simulink model "Openloop_gendata_2015a"  (Simulink 8.5)
settings: Solver=ode45  SolverMode=SingleTasking  StartTime=0.0  StopTime=10  MaxStep=0.001  RelTol=1e-3
settings Model: Creator=manzand  LastModifiedBy=dieman95  CovMetricSettings=dwe  CovHtmlReporting=off  covSaveCumulativeToWorkspaceVar=off  CovSaveSingleToWorkspaceVar=off  CovExternalEMLEnable=on
settings DataIOCC: LimitDataPoints=off  SaveFormat=Dataset  SignalLoggingSaveFormat=Dataset
settings OptimizationCC: ExpressionDepthLimit=128
settings DebuggingCC: UnderspecifiedInitializationDetection=Simplified  MergeDetectMultiDrivingBlocksExec=error  FcnCallInpInsideContextMsg=EnableAllAsError  StateNameClashWarn=none  SFUnexpectedBacktrackingDiag=error  SFNoUnconditionalDefaultTransitionDiag=error
settings HardwareCC: ProdBitPerPointer=64  ProdLargestAtomicFloat=Float  ProdIntDivRoundTo=Zero  ProdEndianess=LittleEndian  ProdHWDeviceType=Specified
settings ModelReferenceCC: PropagateSignalLabelsOutOfModel=on
settings GRTTargetCC: TargetLangStandard=C99 (ISO)  GeneratePreprocessorConditionals=Use local settings  CombineOutputUpdateFcns=on  GRTInterface=off

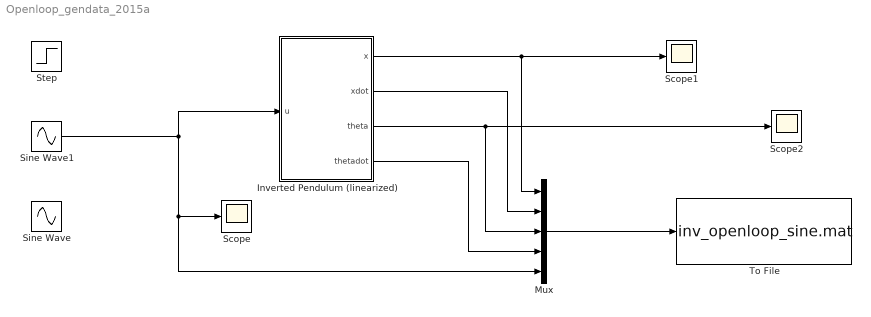
== system Openloop_gendata_2015a ==
  Inverted Pendulum (linearized) : Subsystem
  Mux : Mux  Inputs=5
  Scope : Scope
      settings: TimeRange=auto  MaxDataPoints=5000  SaveToWorkspace=off  SaveName=ScopeData  YMin=-1.25  YMax=1.25  SampleTime=-1
  Scope1 : Scope
      settings: TimeRange=auto  MaxDataPoints=5000  SaveToWorkspace=off  YMin=-49076167611524168.00000  YMax=5452907512391574.00000  SampleTime=-1
  Scope2 : Scope
      settings: TimeRange=auto  MaxDataPoints=5000  SaveToWorkspace=off  SaveName=ScopeData2  YMin=-31802048934758674000.00000  YMax=3533560992750962700.00000  SampleTime=-1
  Sine Wave : Sin  Amplitude=1.4370  Bias=-1.0524  SampleTime=0
  Sine Wave1 : Sin  Amplitude=0.01
  Step : Step  Time=3  SampleTime=0
  To File : ToFile  Filename=inv_openloop_sine.mat  MatrixName=openloop  SampleTime=0.001
      settings: Decimation=2
  wires:
  Sine Wave1/1 -> Inverted Pendulum (linearized)/1(u), Mux/5, Scope/1
  Inverted Pendulum (linearized)/1(x) -> Mux/1, Scope1/1
  Inverted Pendulum (linearized)/3(theta) -> Mux/3, Scope2/1
  Inverted Pendulum (linearized)/2(xdot) -> Mux/2
  Inverted Pendulum (linearized)/4(thetadot) -> Mux/4
  Mux/1 -> To File/1

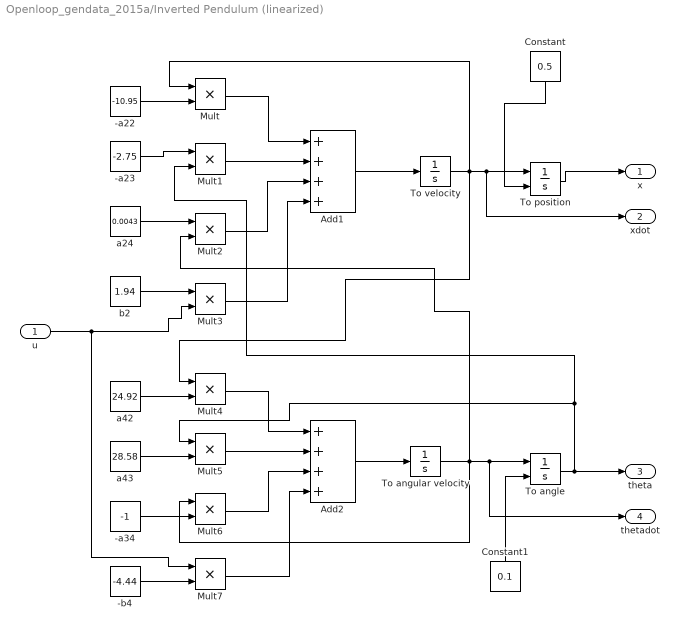
== system Openloop_gendata_2015a/Inverted Pendulum (linearized) ==
  u : Inport
  -a22 : Constant  Value=-10.95
  -a23 : Constant  Value=-2.75
  -a34 : Constant  Value=-1
  -b4 : Constant  Value=-4.44
  Add1 : Sum  Inputs=++++
  Add2 : Sum  Inputs=++++
  Constant : Constant  Value=0.5
  Constant1 : Constant  Value=0.1
  Mult{,1..7} (8 alike) : Product  Inputs=**
  To angle : Integrator  InitialConditionSource=external  InitialCondition=1.5
  To angular velocity : Integrator
  To position : Integrator  InitialConditionSource=external  InitialCondition=1
  To velocity : Integrator
  a24 : Constant  Value=0.0043
  a42 : Constant  Value=24.92
  a43 : Constant  Value=28.58
  b2 : Constant  Value=1.94
  x : Outport
  xdot : Outport  Port=2
  theta : Outport  Port=3
  thetadot : Outport  Port=4
  wires:
  -a22/1 -> Mult/2
  Add2/1 -> To angular velocity/1
  -a34/1 -> Mult6/2
  -b4/1 -> Mult7/2
  Mult6/1 -> Add2/3
  Mult3/1 -> Add1/4
  Mult1/1 -> Add1/2
  Add1/1 -> To velocity/1
  b2/1 -> Mult3/1
  To angular velocity/1 -> Mult6/1, Mult2/2, thetadot/1, To angle/1
  -a23/1 -> Mult1/1
  To velocity/1 -> Mult4/1, Mult/1, xdot/1, To position/1
  To angle/1 -> theta/1, Mult5/1, Mult1/2
  Mult7/1 -> Add2/4
  a43/1 -> Mult5/2
  Mult4/1 -> Add2/1
  Mult2/1 -> Add1/3
  u/1 -> Mult7/1, Mult3/2
  a42/1 -> Mult4/2
  Mult/1 -> Add1/1
  Mult5/1 -> Add2/2
  a24/1 -> Mult2/1
  To position/1 -> x/1
  Constant1/1 -> To angle/2
  Constant/1 -> To position/2
